simulink model "control_filtro_pq_lspyc"  (R2017b)
settings: Solver=ode1  StartTime=0.0  StopTime=0.5  FixedStep=Ts  MaxStep=1e-4  RelTol=1e-3
InitFcn:
  | GlobalParam
values from neighbouring files (symbols this model uses):
  APFon = 0.025    [GlobalParam.m]
  Cdc = 2480e-6    (= 0.00248)    [GlobalParam.m]
  fc = 18000    [GlobalParam.m]
  fe = 50    [GlobalParam.m]
  Ideal = 0    [GlobalParam.m]
  Lf = 0.01    [GlobalParam.m]
  LL = 0.055462    [GlobalParam.m]
  nc = 3    [GlobalParam.m]
  NLLon = 6    [GlobalParam.m]
  Rf = 0.35    [GlobalParam.m]
  RL = 23.232    [GlobalParam.m]
  RLon = 0.0    (= 0)    [GlobalParam.m]
  teta_a = 0    [GlobalParam.m]
  teta_b = -120    [GlobalParam.m]
  teta_c = 120    [GlobalParam.m]
  Tm = 1/fm    (= 5.55555555556e-05)    [GlobalParam.m]
  Ts = 5e-6    (= 5e-06)    [GlobalParam.m]
  Vdc = 63    [GlobalParam.m]
  Vs = 120*sqrt(2)    [GlobalParam.m]
undefined symbols (not defined in the file or in its folder): magnitude
libraries: powerlib x113, simulink x9, powerlib_meascontrol x6, powerlib_extras x5
(part 1 of 2)
settings Model: Creator=user  LastModifiedBy=user
settings OptimizationCC: LifeSpan=inf
settings DebuggingCC: SFExecutionAtInitializationDiag=none
settings CodeAppCC: StateflowObjectComments=on
settings SimscapeCC: SimscapeNormalizeSystem=off

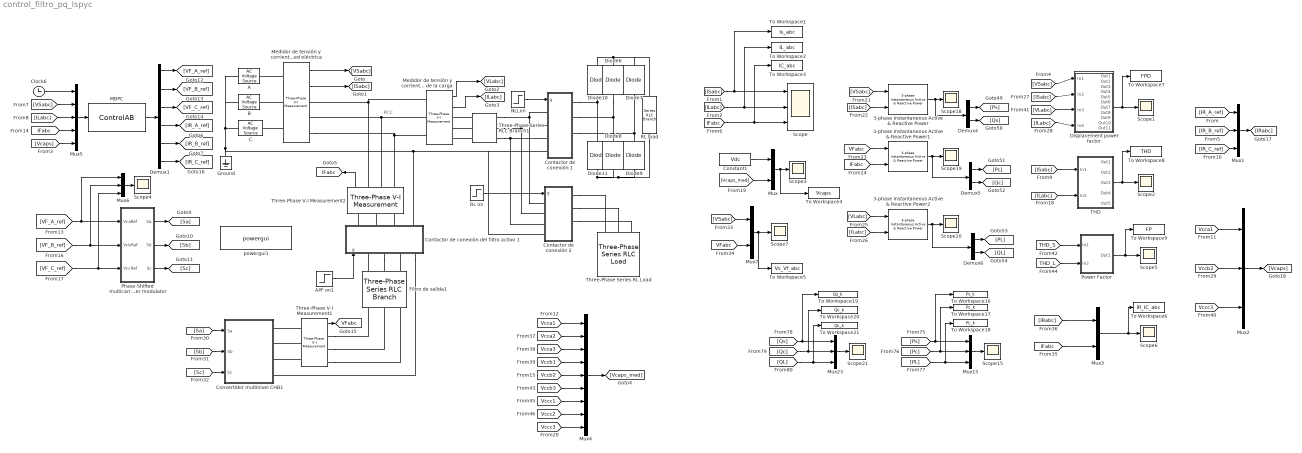
== system control_filtro_pq_lspyc ==
  note: PCC
  " RL load" : powerlib/Elements/Series RLC Branch  LConnTagsString=__new0  RConnTagsString=__new0  BranchType=RL  Resistance=RL*6  Inductance=LL/6  SetiL0=off  InitialCurrent=0  Capacitance=1e-6  Setx0=off  InitialVoltage=0  Measurements=None
  3-phase Instantaneous Active & Reactive Power : powerlib_extras/Measurements/3-phase  Instantaneous  Active & Reactive Power
  3-phase Instantaneous Active & Reactive Power1 : powerlib_extras/Measurements/3-phase  Instantaneous  Active & Reactive Power
  3-phase Instantaneous Active & Reactive Power2 : powerlib_extras/Measurements/3-phase  Instantaneous  Active & Reactive Power
  "A " : powerlib/Electrical Sources/AC Voltage Source  Amplitude=Vs  Phase=teta_a  Frequency=fe  SampleTime=0  Measurements=None  BusType=swing  Pref=10e3  Qref=0  Qmin=-inf  Qmax=+inf
  APF on1 : Step  Time=APFon  SampleTime=0
  "B " : powerlib/Electrical Sources/AC Voltage Source  Amplitude=Vs  Phase=teta_b  Frequency=fe  SampleTime=0  Measurements=None  BusType=swing  Pref=10e3  Qref=0  Qmin=-inf  Qmax=+inf
  "C " : powerlib/Electrical Sources/AC Voltage Source  Amplitude=Vs  Phase=teta_c  Frequency=fe  SampleTime=0  Measurements=None  BusType=swing  Pref=10e3  Qref=0  Qmin=-inf  Qmax=+inf
  Clock6 : Clock
  Constant1 : Constant  Value=Vdc
  Contactor de conexión del filtro activo 1 : Subsystem
  Contactor de conexión 1 : Subsystem
  "Contactor de conexión 2 " : Subsystem
  Convertidor multinivel CHB1 : Subsystem
  Demux1 : Demux  Outputs=6
  Demux4 : Demux  Outputs=2
  Demux5 : Demux  Outputs=2
  Demux6 : Demux  Outputs=2
  Diode{6..11} (6 alike) : powerlib/Power Electronics/Diode  Ron=0.001  Lon=0  Vf=0  IC=0  UseSnubber=off  Rs=500  Cs=250e-9  Measurements=off
  Displacement power factor : Subsystem
  Filtro de salida1 : powerlib/Elements/Three-Phase Series RLC Branch  LConnTagsString=A|B|C  RConnTagsString=A|B|C  BranchType=RL  Resistance=Rf  Inductance=Lf  Capacitance=1e-6  Measurements=None
  Ground : powerlib/Elements/Ground  LConnTagsString=a
  MBPC : MATLABFcn  MATLABFcn=ControlAB  OutputDimensions=6
  Medidor de tensión y corriente de la red eléctrica : powerlib/Measurements/Three-Phase V-I Measurement  VoltageMeasurement=phase-to-ground  SetLabelV=off  LabelV=Vabc  Vpu=off  VpuLL=off  CurrentMeasurement=yes  SetLabelI=off  LabelI=Iabc  Ipu=off  Pbase=100e6  Vbase=500e3  OutputType=Complex  PhasorSimulation=off  PSBequivalent=0
  "Medidor de tensión y corriente de la carga " : powerlib/Measurements/Three-Phase V-I Measurement  VoltageMeasurement=phase-to-ground  SetLabelV=off  LabelV=Vabc  Vpu=off  VpuLL=off  CurrentMeasurement=yes  SetLabelI=off  LabelI=Iabc  Ipu=off  Pbase=100e6  Vbase=500e3  OutputType=Complex  PhasorSimulation=off  PSBequivalent=0
  Mux : Mux  Inputs=2
  Mux{1..2,6,15,23} (5 alike) : Mux  Inputs=3
  Mux3 : Mux  Inputs=2
  Mux4 : Mux  Inputs=9
  Mux5 : Mux  Inputs=5
  Mux7 : Mux  Inputs=2
  "NLLon " : Step  Time=NLLon  SampleTime=0
  Phase-Shifted multicarrier modulator : Subsystem
  "Power Factor " : Subsystem
  "RL on " : Step  Time=RLon  SampleTime=0
  Scope : Scope  NumInputPorts=3
  Scope{1..7,15,18..21} (12 alike) : Scope
  "THD " : Subsystem
  Three-Phase Series RL Load : powerlib/Elements/Three-Phase Series RLC Load  LConnTagsString=A|B|C  Configuration=Y (grounded)  NominalVoltage=120  Vabc=[120 120 120]  Vabcp=[1e3 1e3 1e3]  NominalFrequency=50  UnbalancedPower=on  ActivePower=350/3  InductivePower=833/3  CapacitivePower=0  Pabc=[280 280 280]  QLabc=[200 200 200]  QCabc=[0 0 0]  Pabcp=[10e3 9e3 11e3]  QLabcp=[100 90 110]  QCabcp=[100 90 110]  Measurements=None  LoadType=constant Z
  Three-Phase Series RLC Branch1 : powerlib/Elements/Three-Phase Series RLC Branch  LConnTagsString=A|B|C  RConnTagsString=A|B|C  BranchType=RL  Resistance=0.1  Inductance=0.001  Capacitance=1e-6  Measurements=None
  Three-Phase V-I Measurement1 : powerlib/Measurements/Three-Phase V-I Measurement  VoltageMeasurement=phase-to-ground  SetLabelV=off  LabelV=Vabc  Vpu=off  VpuLL=off  CurrentMeasurement=no  SetLabelI=off  LabelI=Iabc  Ipu=off  Pbase=100e6  Vbase=500e3  OutputType=Complex  PhasorSimulation=off  PSBequivalent=0
  Three-Phase V-I Measurement2 : powerlib/Measurements/Three-Phase V-I Measurement  VoltageMeasurement=no  SetLabelV=off  LabelV=Vabc  Vpu=off  VpuLL=off  CurrentMeasurement=yes  SetLabelI=off  LabelI=Iabc  Ipu=off  Pbase=100e6  Vbase=500e3  OutputType=Complex  PhasorSimulation=off  PSBequivalent=0
  To Workspace1 : ToWorkspace  VariableName=Is_abc  SaveFormat=Timeseries  SampleTime=-1
  To Workspace16 : ToWorkspace  VariableName=Ps_k  SaveFormat=Timeseries  SampleTime=-1
  To Workspace17 : ToWorkspace  VariableName=Pc_k  SaveFormat=Timeseries  SampleTime=-1
  To Workspace18 : ToWorkspace  VariableName=PL_k  SaveFormat=Timeseries  SampleTime=-1
  To Workspace19 : ToWorkspace  VariableName=Qs_k  SaveFormat=Timeseries  SampleTime=-1
  To Workspace2 : ToWorkspace  VariableName=IL_abc  SaveFormat=Timeseries  SampleTime=-1
  To Workspace20 : ToWorkspace  VariableName=Qc_k  SaveFormat=Timeseries  SampleTime=-1
  To Workspace21 : ToWorkspace  VariableName=QL_k  SaveFormat=Timeseries  SampleTime=-1
  To Workspace3 : ToWorkspace  VariableName=IC_abc  SaveFormat=Timeseries  SampleTime=-1
  To Workspace4 : ToWorkspace  VariableName=Vcaps  SaveFormat=Timeseries  SampleTime=-1
  To Workspace5 : ToWorkspace  VariableName=Vs_Vf_abc  SaveFormat=Timeseries  SampleTime=-1
  To Workspace6 : ToWorkspace  VariableName=IR_IC_abc  SaveFormat=Timeseries  SampleTime=-1
  To Workspace7 : ToWorkspace  VariableName=FPD  SaveFormat=Timeseries  SampleTime=-1
  To Workspace8 : ToWorkspace  VariableName=THD  SaveFormat=Timeseries  SampleTime=-1
  To Workspace9 : ToWorkspace  VariableName=FP  SaveFormat=Timeseries  SampleTime=-1
  powergui1 : powerlib/powergui  Priority=1  SimulationMode=Discrete  SampleTime=Ts  frequency=60  Iterations=50  frequencyindice=50  Pbase=100e6  ErrMax=1e-4  UnitsV=kV  UnitsW=MW  buscounter=0  FunctionMessages=off  echomessages=off  EnableUseOfTLC=off  CurrentSourceSwitches=off  DisableSnubberDevices=off  DisableRonSwitches=off  DisableVfSwitches=off  DisplayEquations=off  SolverType=Tustin/Backward Euler (TBE)  Interpol=off  ExternalGateDelay=off  methode=off  Ts=100  x0status=blocks  SPID=on  SwTol=0  HookPort=off  RestoreLinks=warning  ResistiveCurrentMeasurement=off  Frange=[0:2:500]  Ylog=off  Xlog=on  ShowGrid=off  save=off  variable=ZData  structure=ScopeData  ZoomFFT=off  StartTime=0.3  cycles=15  DisplayStyle=1  fundamental=50  FreqAxis=on  MaxFrequency=1500  frequencyindicesteady=1  RmsSteady=1  display=off
  tag scope: IFabc=global, VFabc=global
  wires:
  Medidor de tensión y corriente de la red eléctrica/1 -> [VSabc]
  Medidor de tensión y corriente de la red eléctrica/2 -> [ISabc]
  "Medidor de tensión y corriente de la carga "/2 -> [ILabc]
  [ILabc] -> To Workspace2/1, Scope/2
  Three-Phase V-I Measurement2/1 -> [IFabc]
  Mux5/1 -> MBPC/1
  Clock6/1 -> Mux5/1
  [IFabc] -> To Workspace3/1, Scope/3
  [ISabc] -> To Workspace1/1, Scope/1
  Constant1/1 -> Mux/1
  Mux/1 -> To Workspace4/1, Scope3/1
  Mux6/1 -> Scope4/1
  Phase-Shifted multicarrier modulator/3(Sc) -> [Sc]
  Phase-Shifted multicarrier modulator/1(Sa) -> [Sa]
  [VF_B_ref] -> Mux6/2, Phase-Shifted multicarrier modulator/2(VcbRef)
  [VF_C_ref] -> Mux6/3, Phase-Shifted multicarrier modulator/3(VccRef)
  [VF_A_ref] -> Mux6/1, Phase-Shifted multicarrier modulator/1(VcaRef)
  Phase-Shifted multicarrier modulator/2(Sb) -> [Sb]
  Demux1/1 -> [VF_A_ref]
  Demux1/2 -> [VF_B_ref]
  Demux1/3 -> [VF_C_ref]
  Three-Phase V-I Measurement1/1 -> [VFabc]
  [IFabc] -> Mux3/2
  [IRabc] -> Mux3/1
  [VFabc] -> Mux7/2
  [VSabc] -> Mux7/1
  [Sc] -> Convertidor multinivel CHB1/3(Sc)
  [Sb] -> Convertidor multinivel CHB1/2(Sb)
  Mux3/1 -> To Workspace6/1, Scope6/1
  APF on1/1 -> Contactor de conexión del filtro activo 1/1(g)
  [Sa] -> Convertidor multinivel CHB1/1(Sa)
  Mux7/1 -> To Workspace5/1, Scope7/1
  [Vcaps] -> Mux5/5
  [IFabc] -> Mux5/4
  [ILabc] -> Mux5/3
  [VSabc] -> Mux5/2
  Demux1/4 -> [IR_A_ref]
  Demux1/5 -> [IR_B_ref]
  Demux1/6 -> [IR_C_ref]
  Mux1/1 -> [IRabc]
  [IR_A_ref] -> Mux1/1
  [IR_B_ref] -> Mux1/2
  [IR_C_ref] -> Mux1/3
  Mux2/1 -> [Vcaps]
  [Vcaps_med] -> Mux/2
  MBPC/1 -> Demux1/1
  "RL on "/1 -> "Contactor de conexión 2 "/1(g)
  3-phase Instantaneous Active & Reactive Power/1 -> Scope18/1, Demux4/1
  [VSabc] -> 3-phase Instantaneous Active & Reactive Power/1
  Demux4/2 -> [Qs]
  [ISabc] -> 3-phase Instantaneous Active & Reactive Power/2
  Demux4/1 -> [Ps]
  [IFabc] -> 3-phase Instantaneous Active & Reactive Power1/2
  3-phase Instantaneous Active & Reactive Power1/1 -> Scope19/1, Demux5/1
  [VFabc] -> 3-phase Instantaneous Active & Reactive Power1/1
  Demux5/1 -> [Pc]
  Demux5/2 -> [Qc]
  [VLabc] -> 3-phase Instantaneous Active & Reactive Power2/1
  [ILabc] -> 3-phase Instantaneous Active & Reactive Power2/2
  3-phase Instantaneous Active & Reactive Power2/1 -> Scope20/1, Demux6/1
  Demux6/1 -> [PL]
  Demux6/2 -> [QL]
  Mux15/1 -> Scope15/1
  [Qc] -> Mux23/2, To Workspace20/1
  [PL] -> Mux15/3, To Workspace18/1
  [Ps] -> Mux15/1, To Workspace16/1
  [Pc] -> Mux15/2, To Workspace17/1
  [QL] -> Mux23/3, To Workspace21/1
  Mux23/1 -> Scope21/1
  [Qs] -> Mux23/1, To Workspace19/1
  "Medidor de tensión y corriente de la carga "/1 -> [VLabc]
  "NLLon "/1 -> Contactor de conexión 1/1(g)
  "Power Factor "/1(Out1) -> Scope5/1, To Workspace9/1
  [THD_S] -> "Power Factor "/1(In1)
  [THD_L] -> "Power Factor "/2(In2)
  "THD "/3(Out3) -> Scope2/1, To Workspace8/1
  [ISabc] -> "THD "/1(In1)
  [ILabc] -> "THD "/2(In2)
  Displacement power factor/7(Out7) -> To Workspace7/1, Scope1/1
  [VSabc] -> Displacement power factor/1(In1)
  [ISabc] -> Displacement power factor/2(In2)
  [VLabc] -> Displacement power factor/3(In3)
  [ILabc] -> Displacement power factor/4(In4)
  [Vccc3] -> Mux2/3
  [Vccb2] -> Mux2/2
  [Vcca1] -> Mux2/1
  Mux4/1 -> [Vcaps_med]
  [Vcca1] -> Mux4/1
  [Vcca2] -> Mux4/2
  [Vcca3] -> Mux4/3
  [Vccb1] -> Mux4/4
  [Vccb2] -> Mux4/5
  [Vccb3] -> Mux4/6
  [Vccc1] -> Mux4/7
  [Vccc3] -> Mux4/9
  [Vccc2] -> Mux4/8
  connections:
  Contactor de conexión del filtro activo 1/RConn4 -- Contactor de conexión 1/LConn4 -- "Contactor de conexión 2 "/LConn4 -- "C "/LConn1 -- "A "/LConn1 -- "B "/LConn1 -- Ground/LConn1
  "Medidor de tensión y corriente de la carga "/LConn1 -- Three-Phase V-I Measurement2/RConn1 -- Medidor de tensión y corriente de la red eléctrica/RConn1
  "Medidor de tensión y corriente de la carga "/LConn2 -- Three-Phase V-I Measurement2/RConn2 -- Medidor de tensión y corriente de la red eléctrica/RConn2
  Medidor de tensión y corriente de la red eléctrica/RConn3 -- Three-Phase V-I Measurement2/RConn3 -- "Medidor de tensión y corriente de la carga "/LConn3
  Filtro de salida1/RConn1 -- Contactor de conexión del filtro activo 1/LConn1
  Three-Phase V-I Measurement1/LConn3 -- Convertidor multinivel CHB1/RConn3
  Three-Phase V-I Measurement1/LConn1 -- Convertidor multinivel CHB1/RConn1
  Three-Phase V-I Measurement1/RConn1 -- Filtro de salida1/LConn1
  Contactor de conexión del filtro activo 1/LConn2 -- Filtro de salida1/RConn2
  Three-Phase V-I Measurement1/LConn2 -- Convertidor multinivel CHB1/RConn2
  Filtro de salida1/RConn3 -- Contactor de conexión del filtro activo 1/LConn3
  Contactor de conexión del filtro activo 1/LConn4 -- Convertidor multinivel CHB1/RConn4
  Three-Phase V-I Measurement1/RConn3 -- Filtro de salida1/LConn3
  Three-Phase V-I Measurement1/RConn2 -- Filtro de salida1/LConn2
  Contactor de conexión del filtro activo 1/RConn1 -- Three-Phase V-I Measurement2/LConn1
  Contactor de conexión del filtro activo 1/RConn2 -- Three-Phase V-I Measurement2/LConn2
  Contactor de conexión del filtro activo 1/RConn3 -- Three-Phase V-I Measurement2/LConn3
  Medidor de tensión y corriente de la red eléctrica/LConn3 -- "C "/RConn1
  Medidor de tensión y corriente de la red eléctrica/LConn2 -- "B "/RConn1
  Medidor de tensión y corriente de la red eléctrica/LConn1 -- "A "/RConn1
  "Contactor de conexión 2 "/RConn1 -- Three-Phase Series RL Load/LConn1
  "Contactor de conexión 2 "/RConn2 -- Three-Phase Series RL Load/LConn2
  "Contactor de conexión 2 "/RConn3 -- Three-Phase Series RL Load/LConn3
  Contactor de conexión 1/LConn1 -- Three-Phase Series RLC Branch1/RConn1 -- "Contactor de conexión 2 "/LConn1
  Contactor de conexión 1/LConn2 -- Three-Phase Series RLC Branch1/RConn2 -- "Contactor de conexión 2 "/LConn2
  Contactor de conexión 1/LConn3 -- Three-Phase Series RLC Branch1/RConn3 -- "Contactor de conexión 2 "/LConn3
  Three-Phase Series RLC Branch1/LConn3 -- "Medidor de tensión y corriente de la carga "/RConn3
  Three-Phase Series RLC Branch1/LConn2 -- "Medidor de tensión y corriente de la carga "/RConn2
  Three-Phase Series RLC Branch1/LConn1 -- "Medidor de tensión y corriente de la carga "/RConn1
  Diode10/LConn1 -- Contactor de conexión 1/RConn1 -- Diode11/RConn1
  Diode6/RConn1 -- " RL load"/LConn1 -- Diode7/RConn1 -- Diode10/RConn1
  Diode9/RConn1 -- Contactor de conexión 1/RConn3 -- Diode7/LConn1
  Diode6/LConn1 -- Contactor de conexión 1/RConn2 -- Diode8/RConn1
  Diode11/LConn1 -- " RL load"/RConn1 -- Diode9/LConn1 -- Diode8/LConn1

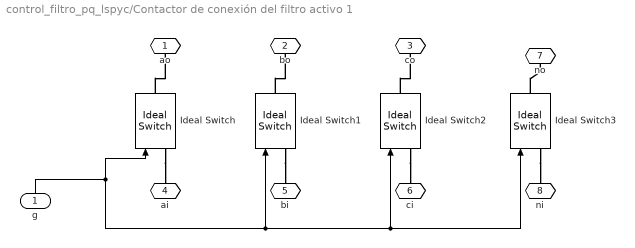
== system control_filtro_pq_lspyc/Contactor de conexión del filtro activo 1 ==
  g : Inport
  Ideal Switch{,1..3} (4 alike) : powerlib/Power Electronics/Ideal Switch  Ron=0.001  Lon=0  IC=0  Rs=1e5  Cs=inf  Measurements=off
  ao : PMIOPort  Port=1  Side=Right
  bo : PMIOPort  Port=2  Side=Right
  co : PMIOPort  Port=3  Side=Right
  ai : PMIOPort  Port=4  Side=Left
  bi : PMIOPort  Port=5  Side=Left
  ci : PMIOPort  Port=6  Side=Left
  no : PMIOPort  Port=7  Side=Left
  ni : PMIOPort  Port=8  Side=Right
  wires:
  g/1 -> Ideal Switch3/1, Ideal Switch2/1, Ideal Switch1/1, Ideal Switch/1
  connections:
  Ideal Switch1/RConn1 -- bo/RConn1
  Ideal Switch1/LConn1 -- bi/RConn1
  Ideal Switch/RConn1 -- ao/RConn1
  Ideal Switch2/RConn1 -- co/RConn1
  Ideal Switch2/LConn1 -- ci/RConn1
  Ideal Switch/LConn1 -- ai/RConn1
  Ideal Switch3/LConn1 -- ni/RConn1
  Ideal Switch3/RConn1 -- no/RConn1

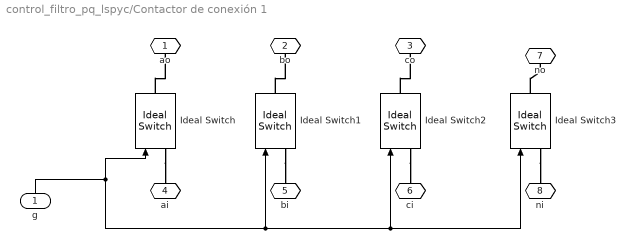
== system control_filtro_pq_lspyc/Contactor de conexión 1 ==
  g : Inport
  Ideal Switch{,1..3} (4 alike) : powerlib/Power Electronics/Ideal Switch  Ron=0.001  Lon=0  IC=0  Rs=1e5  Cs=inf  Measurements=off
  ao : PMIOPort  Port=1  Side=Right
  bo : PMIOPort  Port=2  Side=Right
  co : PMIOPort  Port=3  Side=Right
  ai : PMIOPort  Port=4  Side=Left
  bi : PMIOPort  Port=5  Side=Left
  ci : PMIOPort  Port=6  Side=Left
  no : PMIOPort  Port=7  Side=Left
  ni : PMIOPort  Port=8  Side=Right
  wires:
  g/1 -> Ideal Switch3/1, Ideal Switch2/1, Ideal Switch1/1, Ideal Switch/1
  connections:
  Ideal Switch1/RConn1 -- bo/RConn1
  Ideal Switch1/LConn1 -- bi/RConn1
  Ideal Switch/RConn1 -- ao/RConn1
  Ideal Switch2/RConn1 -- co/RConn1
  Ideal Switch2/LConn1 -- ci/RConn1
  Ideal Switch/LConn1 -- ai/RConn1
  Ideal Switch3/LConn1 -- ni/RConn1
  Ideal Switch3/RConn1 -- no/RConn1

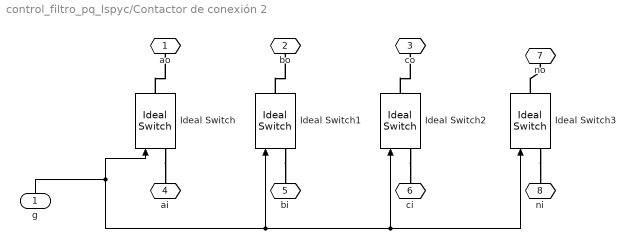
== system control_filtro_pq_lspyc/Contactor de conexión 2  ==
  g : Inport
  Ideal Switch{,1..3} (4 alike) : powerlib/Power Electronics/Ideal Switch  Ron=0.001  Lon=0  IC=0  Rs=1e5  Cs=inf  Measurements=off
  ao : PMIOPort  Port=1  Side=Right
  bo : PMIOPort  Port=2  Side=Right
  co : PMIOPort  Port=3  Side=Right
  ai : PMIOPort  Port=4  Side=Left
  bi : PMIOPort  Port=5  Side=Left
  ci : PMIOPort  Port=6  Side=Left
  no : PMIOPort  Port=7  Side=Left
  ni : PMIOPort  Port=8  Side=Right
  wires:
  g/1 -> Ideal Switch3/1, Ideal Switch2/1, Ideal Switch1/1, Ideal Switch/1
  connections:
  Ideal Switch1/RConn1 -- bo/RConn1
  Ideal Switch1/LConn1 -- bi/RConn1
  Ideal Switch/RConn1 -- ao/RConn1
  Ideal Switch2/RConn1 -- co/RConn1
  Ideal Switch2/LConn1 -- ci/RConn1
  Ideal Switch/LConn1 -- ai/RConn1
  Ideal Switch3/LConn1 -- ni/RConn1
  Ideal Switch3/RConn1 -- no/RConn1

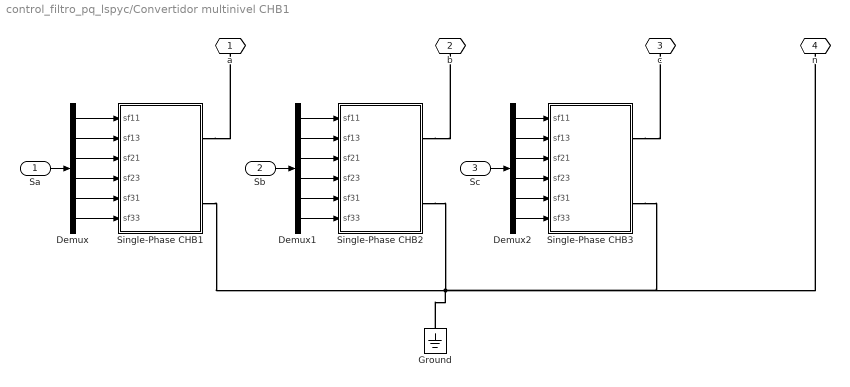
== system control_filtro_pq_lspyc/Convertidor multinivel CHB1 ==
  Sa : Inport
  Sb : Inport  Port=2
  Sc : Inport  Port=3
  Demux : Demux  Outputs=6
  Demux1 : Demux  Outputs=6
  Demux2 : Demux  Outputs=6
  Ground : powerlib/Elements/Ground  LConnTagsString=a
  Single-Phase CHB1 : Subsystem
  Single-Phase CHB2 : Subsystem
  Single-Phase CHB3 : Subsystem
  a : PMIOPort  Port=1  Side=Right
  b : PMIOPort  Port=2  Side=Right
  c : PMIOPort  Port=3  Side=Right
  n : PMIOPort  Port=4  Side=Right
  wires:
  Demux/4 -> Single-Phase CHB1/4(sf23)
  Demux/6 -> Single-Phase CHB1/6(sf33)
  Demux/3 -> Single-Phase CHB1/3(sf21)
  Demux/2 -> Single-Phase CHB1/2(sf13)
  Demux/1 -> Single-Phase CHB1/1(sf11)
  Demux1/3 -> Single-Phase CHB2/3(sf21)
  Sa/1 -> Demux/1
  Sb/1 -> Demux1/1
  Sc/1 -> Demux2/1
  Demux2/1 -> Single-Phase CHB3/1(sf11)
  Demux1/1 -> Single-Phase CHB2/1(sf11)
  Demux1/6 -> Single-Phase CHB2/6(sf33)
  Demux2/6 -> Single-Phase CHB3/6(sf33)
  Demux/5 -> Single-Phase CHB1/5(sf31)
  Demux1/2 -> Single-Phase CHB2/2(sf13)
  Demux2/5 -> Single-Phase CHB3/5(sf31)
  Demux1/4 -> Single-Phase CHB2/4(sf23)
  Demux2/4 -> Single-Phase CHB3/4(sf23)
  Demux1/5 -> Single-Phase CHB2/5(sf31)
  Demux2/3 -> Single-Phase CHB3/3(sf21)
  Demux2/2 -> Single-Phase CHB3/2(sf13)
  connections:
  Single-Phase CHB2/RConn1 -- b/RConn1
  Single-Phase CHB1/RConn2 -- Ground/LConn1 -- Single-Phase CHB2/RConn2 -- Single-Phase CHB3/RConn2 -- n/RConn1
  Single-Phase CHB1/RConn1 -- a/RConn1
  Single-Phase CHB3/RConn1 -- c/RConn1

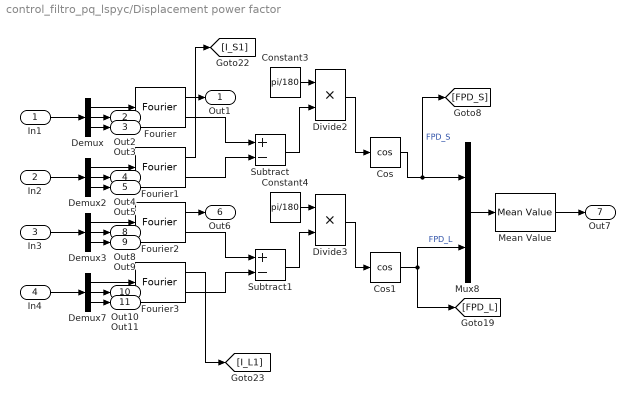
== system control_filtro_pq_lspyc/Displacement power factor ==
  In1 : Inport
  In2 : Inport  Port=2
  In3 : Inport  Port=3
  In4 : Inport  Port=4
  Constant3 : Constant  Value=pi/180
  Constant4 : Constant  Value=pi/180
  Cos : Trigonometry  Operator=cos
  Cos1 : Trigonometry  Operator=cos
  Demux{,2..3,7} (4 alike) : Demux  Outputs=3
  Divide2 : Product  Inputs=**
  Divide3 : Product  Inputs=**
  Fourier{,1..3} (4 alike) : powerlib_meascontrol/Measurements/Fourier  Freq=60  n=1  InInit=[0, 0]  Ts=0
      settings: SourceProductName=Simscape Power Systems
  Mean Value : powerlib_extras/Measurements/Mean Value  Period=1/100
  Mux8 : Mux  Inputs=2
  Subtract : Sum  Inputs=+-
  Subtract1 : Sum  Inputs=+-
  Out1 : Outport
  Out2 : Outport  Port=2
  Out3 : Outport  Port=3
  Out4 : Outport  Port=4
  Out5 : Outport  Port=5
  Out6 : Outport  Port=6
  Out7 : Outport  Port=7
  Out8 : Outport  Port=8
  Out9 : Outport  Port=9
  Out10 : Outport  Port=10
  Out11 : Outport  Port=11
  wires:
  Demux/3 -> Out3/1
  Fourier2/1 -> Out6/1
  Demux/2 -> Out2/1
  Demux7/2 -> Out10/1
  Demux3/2 -> Out8/1
  Fourier/1 -> Out1/1
  Demux7/3 -> Out11/1
  Demux3/3 -> Out9/1
  Fourier3/2 -> Subtract1/2
  Mux8/1 -> Mean Value/1
  Demux2/1 -> Fourier1/1
  In1/1 -> Demux/1
  Constant3/1 -> Divide2/1
  Fourier1/1 -> [I_S1]
  Subtract/1 -> Divide2/2
  Fourier2/2 -> Subtract1/1
  Cos/1 -> Mux8/1, [FPD_S]  "FPD_S"
  Demux/1 -> Fourier/1
  Mean Value/1 -> Out7/1
  Demux3/1 -> Fourier2/1
  Divide3/1 -> Cos1/1
  Fourier1/2 -> Subtract/2
  Constant4/1 -> Divide3/1
  In2/1 -> Demux2/1
  Fourier/2 -> Subtract/1
  Demux7/1 -> Fourier3/1
  Cos1/1 -> Mux8/2, [FPD_L]  "FPD_L"
  In3/1 -> Demux3/1
  In4/1 -> Demux7/1
  Subtract1/1 -> Divide3/2
  Fourier3/1 -> [I_L1]
  Divide2/1 -> Cos/1
  Demux2/2 -> Out4/1
  Demux2/3 -> Out5/1

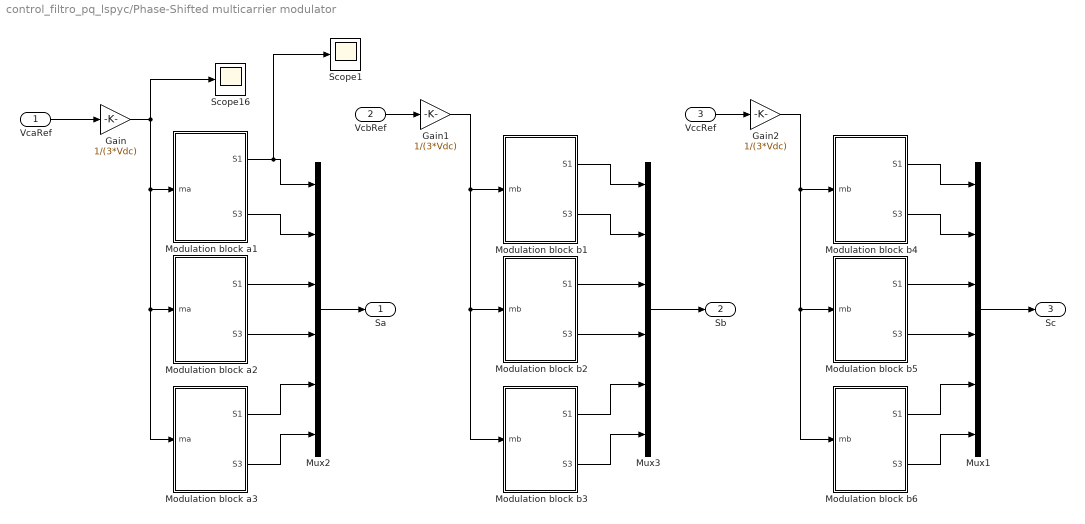
== system control_filtro_pq_lspyc/Phase-Shifted multicarrier modulator ==
  VcaRef : Inport
  VcbRef : Inport  Port=2
  VccRef : Inport  Port=3
  Gain : Gain  Gain=1/(3*Vdc)
  Gain1 : Gain  Gain=1/(3*Vdc)
  Gain2 : Gain  Gain=1/(3*Vdc)
  Modulation block a1 : Subsystem
  Modulation block a2 : Subsystem
  Modulation block a3 : Subsystem
  Modulation block b1 : Subsystem
  Modulation block b2 : Subsystem
  Modulation block b3 : Subsystem
  Modulation block b4 : Subsystem
  Modulation block b5 : Subsystem
  Modulation block b6 : Subsystem
  Mux1 : Mux  Inputs=6
  Mux2 : Mux  Inputs=6
  Mux3 : Mux  Inputs=6
  Scope1 : Scope
  Scope16 : Scope
  Sa : Outport
  Sb : Outport  Port=2
  Sc : Outport  Port=3
  wires:
  Gain1/1 -> Modulation block b1/1(mb), Modulation block b2/1(mb), Modulation block b3/1(mb)
  Gain/1 -> Modulation block a1/1(ma), Modulation block a3/1(ma), Modulation block a2/1(ma), Scope16/1
  Modulation block a2/2(S3) -> Mux2/4
  Modulation block a2/1(S1) -> Mux2/3
  Modulation block a3/1(S1) -> Mux2/5
  Modulation block a3/2(S3) -> Mux2/6
  Modulation block a1/2(S3) -> Mux2/2
  Mux2/1 -> Sa/1
  Modulation block b2/2(S3) -> Mux3/4
  Modulation block b3/1(S1) -> Mux3/5
  Modulation block b3/2(S3) -> Mux3/6
  Modulation block b2/1(S1) -> Mux3/3
  Modulation block b1/2(S3) -> Mux3/2
  Modulation block b1/1(S1) -> Mux3/1
  Mux3/1 -> Sb/1
  VcbRef/1 -> Gain1/1
  VccRef/1 -> Gain2/1
  VcaRef/1 -> Gain/1
  Modulation block a1/1(S1) -> Scope1/1, Mux2/1
  Gain2/1 -> Modulation block b4/1(mb), Modulation block b5/1(mb), Modulation block b6/1(mb)
  Modulation block b4/2(S3) -> Mux1/2
  Modulation block b4/1(S1) -> Mux1/1
  Mux1/1 -> Sc/1
  Modulation block b5/1(S1) -> Mux1/3
  Modulation block b6/2(S3) -> Mux1/6
  Modulation block b6/1(S1) -> Mux1/5
  Modulation block b5/2(S3) -> Mux1/4

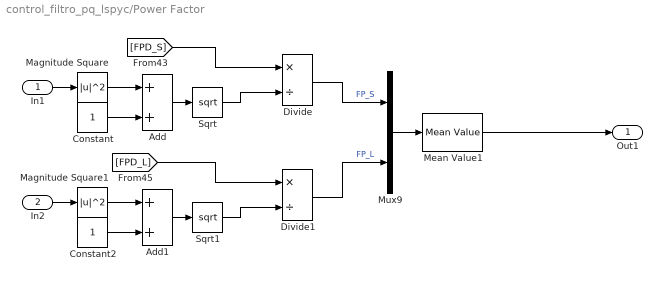
== system control_filtro_pq_lspyc/Power Factor  ==
  In1 : Inport
  In2 : Inport  Port=2
  Add : Sum
  Add1 : Sum
  Constant : Constant
  Constant2 : Constant
  Divide : Product  Inputs=*/
  Divide1 : Product  Inputs=*/
  Magnitude Square : Math  Operator=magnitude^2  RndMeth=Zero  SaturateOnIntegerOverflow=on
  Magnitude Square1 : Math  Operator=magnitude^2  RndMeth=Zero  SaturateOnIntegerOverflow=on
  Mean Value1 : powerlib_extras/Measurements/Mean Value  Period=1/100
  Mux9 : Mux  Inputs=2
  Sqrt : Sqrt  SaturateOnIntegerOverflow=on
  Sqrt1 : Sqrt  SaturateOnIntegerOverflow=on
  Out1 : Outport
  wires:
  In1/1 -> Magnitude Square/1
  Magnitude Square/1 -> Add/1
  Divide1/1 -> Mux9/2  "FP_L"
  Constant/1 -> Add/2
  Mux9/1 -> Mean Value1/1
  Sqrt/1 -> Divide/2
  [FPD_L] -> Divide1/1
  [FPD_S] -> Divide/1
  Add1/1 -> Sqrt1/1
  Add/1 -> Sqrt/1
  In2/1 -> Magnitude Square1/1
  Constant2/1 -> Add1/2
  Sqrt1/1 -> Divide1/2
  Magnitude Square1/1 -> Add1/1
  Divide/1 -> Mux9/1  "FP_S"
  Mean Value1/1 -> Out1/1

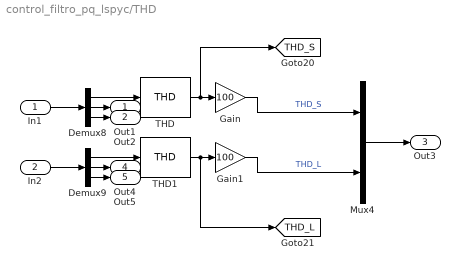
== system control_filtro_pq_lspyc/THD  ==
  In1 : Inport
  In2 : Inport  Port=2
  Demux8 : Demux  Outputs=3
  Demux9 : Demux  Outputs=3
  Gain : Gain  Gain=100
  Gain1 : Gain  Gain=100
  Mux4 : Mux  Inputs=2
  THD : powerlib_meascontrol/Measurements/THD  Freq=50  Ts=Ts
  THD1 : powerlib_meascontrol/Measurements/THD  Freq=50  Ts=Ts
  Out1 : Outport
  Out2 : Outport  Port=2
  Out3 : Outport  Port=3
  Out4 : Outport  Port=4
  Out5 : Outport  Port=5
  tag scope: THD_L=global, THD_S=global
  wires:
  Demux8/1 -> THD/1
  Gain1/1 -> Mux4/2  "THD_L"
  Mux4/1 -> Out3/1
  Gain/1 -> Mux4/1  "THD_S"
  In2/1 -> Demux9/1
  THD1/1 -> [THD_L], Gain1/1
  Demux9/1 -> THD1/1
  In1/1 -> Demux8/1
  THD/1 -> [THD_S], Gain/1
  Demux8/3 -> Out2/1
  Demux8/2 -> Out1/1
  Demux9/2 -> Out4/1
  Demux9/3 -> Out5/1

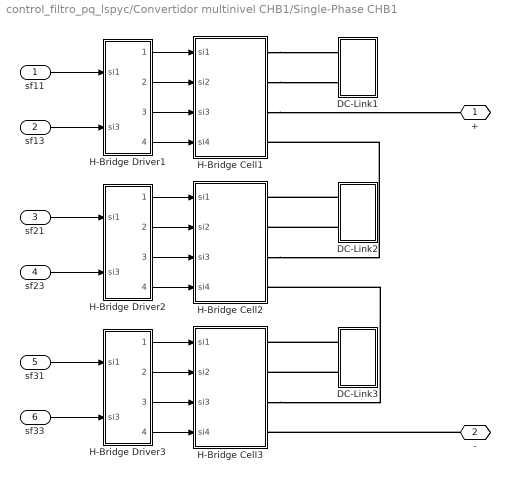
== system control_filtro_pq_lspyc/Convertidor multinivel CHB1/Single-Phase CHB1 ==
  sf11 : Inport
  sf13 : Inport  Port=2
  sf21 : Inport  Port=3
  sf23 : Inport  Port=4
  sf31 : Inport  Port=5
  sf33 : Inport  Port=6
  DC-Link1 : Subsystem
  DC-Link2 : Subsystem
  DC-Link3 : Subsystem
  H-Bridge Cell1 : Subsystem
  H-Bridge Cell2 : Subsystem
  H-Bridge Cell3 : Subsystem
  H-Bridge Driver1 : Subsystem
  H-Bridge Driver2 : Subsystem
  H-Bridge Driver3 : Subsystem
  + : PMIOPort  Port=1  Side=Right
  - : PMIOPort  Port=2  Side=Right
  wires:
  H-Bridge Driver2/1(1) -> H-Bridge Cell2/1(si1)
  H-Bridge Driver2/3(3) -> H-Bridge Cell2/3(si3)
  H-Bridge Driver2/2(2) -> H-Bridge Cell2/2(si2)
  H-Bridge Driver2/4(4) -> H-Bridge Cell2/4(si4)
  H-Bridge Driver1/1(1) -> H-Bridge Cell1/1(si1)
  H-Bridge Driver1/2(2) -> H-Bridge Cell1/2(si2)
  H-Bridge Driver1/3(3) -> H-Bridge Cell1/3(si3)
  H-Bridge Driver1/4(4) -> H-Bridge Cell1/4(si4)
  sf23/1 -> H-Bridge Driver2/2(si3)
  sf13/1 -> H-Bridge Driver1/2(si3)
  sf21/1 -> H-Bridge Driver2/1(si1)
  sf31/1 -> H-Bridge Driver3/1(si1)
  sf11/1 -> H-Bridge Driver1/1(si1)
  sf33/1 -> H-Bridge Driver3/2(si3)
  H-Bridge Driver3/2(2) -> H-Bridge Cell3/2(si2)
  H-Bridge Driver3/1(1) -> H-Bridge Cell3/1(si1)
  H-Bridge Driver3/3(3) -> H-Bridge Cell3/3(si3)
  H-Bridge Driver3/4(4) -> H-Bridge Cell3/4(si4)
  connections:
  H-Bridge Cell2/RConn3 -- H-Bridge Cell1/RConn4
  DC-Link2/RConn2 -- H-Bridge Cell2/RConn2
  DC-Link2/RConn1 -- H-Bridge Cell2/RConn1
  H-Bridge Cell1/RConn1 -- DC-Link1/RConn1
  H-Bridge Cell1/RConn2 -- DC-Link1/RConn2
  H-Bridge Cell1/RConn3 -- +/RConn1
  -/RConn1 -- H-Bridge Cell3/RConn4
  H-Bridge Cell3/RConn3 -- H-Bridge Cell2/RConn4
  DC-Link3/RConn2 -- H-Bridge Cell3/RConn2
  DC-Link3/RConn1 -- H-Bridge Cell3/RConn1

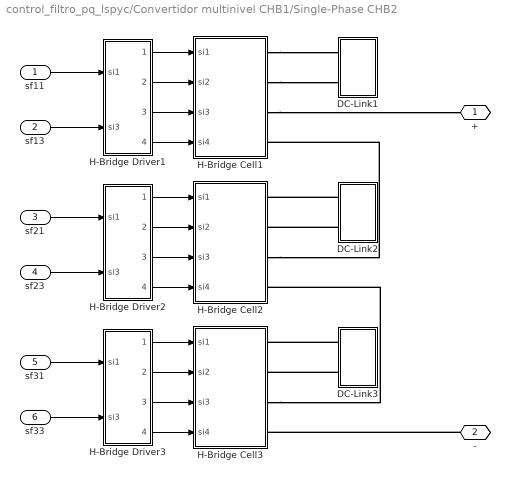
== system control_filtro_pq_lspyc/Convertidor multinivel CHB1/Single-Phase CHB2 ==
  sf11 : Inport
  sf13 : Inport  Port=2
  sf21 : Inport  Port=3
  sf23 : Inport  Port=4
  sf31 : Inport  Port=5
  sf33 : Inport  Port=6
  DC-Link1 : Subsystem
  DC-Link2 : Subsystem
  DC-Link3 : Subsystem
  H-Bridge Cell1 : Subsystem
  H-Bridge Cell2 : Subsystem
  H-Bridge Cell3 : Subsystem
  H-Bridge Driver1 : Subsystem
  H-Bridge Driver2 : Subsystem
  H-Bridge Driver3 : Subsystem
  + : PMIOPort  Port=1  Side=Right
  - : PMIOPort  Port=2  Side=Right
  wires:
  H-Bridge Driver2/1(1) -> H-Bridge Cell2/1(si1)
  H-Bridge Driver2/3(3) -> H-Bridge Cell2/3(si3)
  H-Bridge Driver2/2(2) -> H-Bridge Cell2/2(si2)
  H-Bridge Driver2/4(4) -> H-Bridge Cell2/4(si4)
  H-Bridge Driver1/1(1) -> H-Bridge Cell1/1(si1)
  H-Bridge Driver1/2(2) -> H-Bridge Cell1/2(si2)
  H-Bridge Driver1/3(3) -> H-Bridge Cell1/3(si3)
  H-Bridge Driver1/4(4) -> H-Bridge Cell1/4(si4)
  sf23/1 -> H-Bridge Driver2/2(si3)
  sf13/1 -> H-Bridge Driver1/2(si3)
  sf21/1 -> H-Bridge Driver2/1(si1)
  sf31/1 -> H-Bridge Driver3/1(si1)
  sf11/1 -> H-Bridge Driver1/1(si1)
  sf33/1 -> H-Bridge Driver3/2(si3)
  H-Bridge Driver3/2(2) -> H-Bridge Cell3/2(si2)
  H-Bridge Driver3/1(1) -> H-Bridge Cell3/1(si1)
  H-Bridge Driver3/3(3) -> H-Bridge Cell3/3(si3)
  H-Bridge Driver3/4(4) -> H-Bridge Cell3/4(si4)
  connections:
  H-Bridge Cell2/RConn3 -- H-Bridge Cell1/RConn4
  DC-Link2/RConn2 -- H-Bridge Cell2/RConn2
  DC-Link2/RConn1 -- H-Bridge Cell2/RConn1
  H-Bridge Cell1/RConn1 -- DC-Link1/RConn1
  H-Bridge Cell1/RConn2 -- DC-Link1/RConn2
  H-Bridge Cell1/RConn3 -- +/RConn1
  -/RConn1 -- H-Bridge Cell3/RConn4
  H-Bridge Cell3/RConn3 -- H-Bridge Cell2/RConn4
  DC-Link3/RConn2 -- H-Bridge Cell3/RConn2
  DC-Link3/RConn1 -- H-Bridge Cell3/RConn1

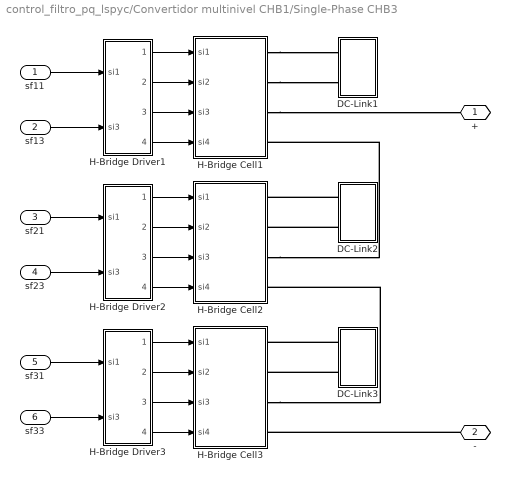
== system control_filtro_pq_lspyc/Convertidor multinivel CHB1/Single-Phase CHB3 ==
  sf11 : Inport
  sf13 : Inport  Port=2
  sf21 : Inport  Port=3
  sf23 : Inport  Port=4
  sf31 : Inport  Port=5
  sf33 : Inport  Port=6
  DC-Link1 : Subsystem
  DC-Link2 : Subsystem
  DC-Link3 : Subsystem
  H-Bridge Cell1 : Subsystem
  H-Bridge Cell2 : Subsystem
  H-Bridge Cell3 : Subsystem
  H-Bridge Driver1 : Subsystem
  H-Bridge Driver2 : Subsystem
  H-Bridge Driver3 : Subsystem
  + : PMIOPort  Port=1  Side=Right
  - : PMIOPort  Port=2  Side=Right
  wires:
  H-Bridge Driver2/1(1) -> H-Bridge Cell2/1(si1)
  H-Bridge Driver2/3(3) -> H-Bridge Cell2/3(si3)
  H-Bridge Driver2/2(2) -> H-Bridge Cell2/2(si2)
  H-Bridge Driver2/4(4) -> H-Bridge Cell2/4(si4)
  H-Bridge Driver1/1(1) -> H-Bridge Cell1/1(si1)
  H-Bridge Driver1/2(2) -> H-Bridge Cell1/2(si2)
  H-Bridge Driver1/3(3) -> H-Bridge Cell1/3(si3)
  H-Bridge Driver1/4(4) -> H-Bridge Cell1/4(si4)
  sf23/1 -> H-Bridge Driver2/2(si3)
  sf13/1 -> H-Bridge Driver1/2(si3)
  sf21/1 -> H-Bridge Driver2/1(si1)
  sf31/1 -> H-Bridge Driver3/1(si1)
  sf11/1 -> H-Bridge Driver1/1(si1)
  sf33/1 -> H-Bridge Driver3/2(si3)
  H-Bridge Driver3/2(2) -> H-Bridge Cell3/2(si2)
  H-Bridge Driver3/1(1) -> H-Bridge Cell3/1(si1)
  H-Bridge Driver3/3(3) -> H-Bridge Cell3/3(si3)
  H-Bridge Driver3/4(4) -> H-Bridge Cell3/4(si4)
  connections:
  H-Bridge Cell2/RConn3 -- H-Bridge Cell1/RConn4
  DC-Link2/RConn2 -- H-Bridge Cell2/RConn2
  DC-Link2/RConn1 -- H-Bridge Cell2/RConn1
  H-Bridge Cell1/RConn1 -- DC-Link1/RConn1
  H-Bridge Cell1/RConn2 -- DC-Link1/RConn2
  H-Bridge Cell1/RConn3 -- +/RConn1
  -/RConn1 -- H-Bridge Cell3/RConn4
  H-Bridge Cell3/RConn3 -- H-Bridge Cell2/RConn4
  DC-Link3/RConn2 -- H-Bridge Cell3/RConn2
  DC-Link3/RConn1 -- H-Bridge Cell3/RConn1

== system control_filtro_pq_lspyc/Phase-Shifted multicarrier modulator/Modulation block a1 ==
  ma : Inport
  Data Type Conversion : DataTypeConversion  OutDataTypeStr=double
  Data Type Conversion3 : DataTypeConversion  OutDataTypeStr=double
  Gain1 : Gain  Gain=-1
  Relational Operator : RelationalOperator  Operator=<=  OutDataTypeStr=boolean  RndMeth=Nearest
  Relational Operator2 : RelationalOperator  Operator=<=  OutDataTypeStr=boolean  RndMeth=Nearest
  Repeating Sequence1 : simulink/Sources/Repeating Sequence  rep_seq_t="[0 (1/fc)/2  1/fc]"  rep_seq_y=[-1 1 -1]
  Scope : Scope
  S1 : Outport
  S3 : Outport  Port=2
  wires:
  Relational Operator/1 -> Data Type Conversion/1
  Repeating Sequence1/1 -> Scope/1, Relational Operator/1, Relational Operator2/1
  Data Type Conversion/1 -> S1/1
  ma/1 -> Relational Operator/2, Gain1/1
  Relational Operator2/1 -> Data Type Conversion3/1
  Data Type Conversion3/1 -> S3/1
  Gain1/1 -> Relational Operator2/2

== system control_filtro_pq_lspyc/Phase-Shifted multicarrier modulator/Modulation block a2 ==
  ma : Inport
  Data Type Conversion : DataTypeConversion  OutDataTypeStr=double
  Data Type Conversion3 : DataTypeConversion  OutDataTypeStr=double
  Gain1 : Gain  Gain=-1
  Relational Operator : RelationalOperator  Operator=<=  OutDataTypeStr=boolean  RndMeth=Nearest
  Relational Operator2 : RelationalOperator  Operator=<=  OutDataTypeStr=boolean  RndMeth=Nearest
  Repeating Sequence1 : simulink/Sources/Repeating Sequence  rep_seq_t="[0 (1/fc)/2  1/fc]"  rep_seq_y=[-1 1 -1]
  Transport Delay : TransportDelay  DelayTime=Tm*(180/nc)/360
  S1 : Outport
  S3 : Outport  Port=2
  wires:
  Relational Operator/1 -> Data Type Conversion/1
  Repeating Sequence1/1 -> Transport Delay/1
  Data Type Conversion/1 -> S1/1
  ma/1 -> Relational Operator/2, Gain1/1
  Relational Operator2/1 -> Data Type Conversion3/1
  Data Type Conversion3/1 -> S3/1
  Gain1/1 -> Relational Operator2/2
  Transport Delay/1 -> Relational Operator/1, Relational Operator2/1

== system control_filtro_pq_lspyc/Phase-Shifted multicarrier modulator/Modulation block a3 ==
  ma : Inport
  Data Type Conversion : DataTypeConversion  OutDataTypeStr=double
  Data Type Conversion3 : DataTypeConversion  OutDataTypeStr=double
  Gain1 : Gain  Gain=-1
  Relational Operator : RelationalOperator  Operator=<=  OutDataTypeStr=boolean  RndMeth=Nearest
  Relational Operator2 : RelationalOperator  Operator=<=  OutDataTypeStr=boolean  RndMeth=Nearest
  Repeating Sequence1 : simulink/Sources/Repeating Sequence  rep_seq_t="[0 (1/fc)/2  1/fc]"  rep_seq_y=[-1 1 -1]
  Transport Delay : TransportDelay  DelayTime=(Tm*(180/nc)/360)*2
  S1 : Outport
  S3 : Outport  Port=2
  wires:
  Relational Operator/1 -> Data Type Conversion/1
  Repeating Sequence1/1 -> Transport Delay/1
  Data Type Conversion/1 -> S1/1
  ma/1 -> Relational Operator/2, Gain1/1
  Relational Operator2/1 -> Data Type Conversion3/1
  Data Type Conversion3/1 -> S3/1
  Gain1/1 -> Relational Operator2/2
  Transport Delay/1 -> Relational Operator/1, Relational Operator2/1

== system control_filtro_pq_lspyc/Phase-Shifted multicarrier modulator/Modulation block b1 ==
  mb : Inport
  Data Type Conversion : DataTypeConversion  OutDataTypeStr=double
  Data Type Conversion3 : DataTypeConversion  OutDataTypeStr=double
  Gain1 : Gain  Gain=-1
  Relational Operator : RelationalOperator  Operator=<=  OutDataTypeStr=boolean  RndMeth=Nearest
  Relational Operator2 : RelationalOperator  Operator=<=  OutDataTypeStr=boolean  RndMeth=Nearest
  Repeating Sequence1 : simulink/Sources/Repeating Sequence  rep_seq_t="[0 (1/fc)/2  1/fc]"  rep_seq_y=[-1 1 -1]
  S1 : Outport
  S3 : Outport  Port=2
  wires:
  Relational Operator/1 -> Data Type Conversion/1
  Repeating Sequence1/1 -> Relational Operator/1, Relational Operator2/1
  Data Type Conversion/1 -> S1/1
  mb/1 -> Relational Operator/2, Gain1/1
  Relational Operator2/1 -> Data Type Conversion3/1
  Data Type Conversion3/1 -> S3/1
  Gain1/1 -> Relational Operator2/2

== system control_filtro_pq_lspyc/Phase-Shifted multicarrier modulator/Modulation block b2 ==
  mb : Inport
  Data Type Conversion : DataTypeConversion  OutDataTypeStr=double
  Data Type Conversion3 : DataTypeConversion  OutDataTypeStr=double
  Gain1 : Gain  Gain=-1
  Relational Operator : RelationalOperator  Operator=<=  OutDataTypeStr=boolean  RndMeth=Nearest
  Relational Operator2 : RelationalOperator  Operator=<=  OutDataTypeStr=boolean  RndMeth=Nearest
  Repeating Sequence1 : simulink/Sources/Repeating Sequence  rep_seq_t="[0 (1/fc)/2  1/fc]"  rep_seq_y=[-1 1 -1]
  Transport Delay : TransportDelay  DelayTime=Tm*(180/nc)/360
  S1 : Outport
  S3 : Outport  Port=2
  wires:
  Relational Operator/1 -> Data Type Conversion/1
  Repeating Sequence1/1 -> Transport Delay/1
  Data Type Conversion/1 -> S1/1
  mb/1 -> Relational Operator/2, Gain1/1
  Relational Operator2/1 -> Data Type Conversion3/1
  Data Type Conversion3/1 -> S3/1
  Gain1/1 -> Relational Operator2/2
  Transport Delay/1 -> Relational Operator/1, Relational Operator2/1

== system control_filtro_pq_lspyc/Phase-Shifted multicarrier modulator/Modulation block b3 ==
  mb : Inport
  Data Type Conversion : DataTypeConversion  OutDataTypeStr=double
  Data Type Conversion3 : DataTypeConversion  OutDataTypeStr=double
  Gain1 : Gain  Gain=-1
  Relational Operator : RelationalOperator  Operator=<=  OutDataTypeStr=boolean  RndMeth=Nearest
  Relational Operator2 : RelationalOperator  Operator=<=  OutDataTypeStr=boolean  RndMeth=Nearest
  Repeating Sequence1 : simulink/Sources/Repeating Sequence  rep_seq_t="[0 (1/fc)/2  1/fc]"  rep_seq_y=[-1 1 -1]
  Transport Delay : TransportDelay  DelayTime=(Tm*(180/nc)/360)*2
  S1 : Outport
  S3 : Outport  Port=2
  wires:
  Relational Operator/1 -> Data Type Conversion/1
  Repeating Sequence1/1 -> Transport Delay/1
  Data Type Conversion/1 -> S1/1
  mb/1 -> Relational Operator/2, Gain1/1
  Relational Operator2/1 -> Data Type Conversion3/1
  Data Type Conversion3/1 -> S3/1
  Gain1/1 -> Relational Operator2/2
  Transport Delay/1 -> Relational Operator/1, Relational Operator2/1

== system control_filtro_pq_lspyc/Phase-Shifted multicarrier modulator/Modulation block b4 ==
  mb : Inport
  Data Type Conversion : DataTypeConversion  OutDataTypeStr=double
  Data Type Conversion3 : DataTypeConversion  OutDataTypeStr=double
  Gain1 : Gain  Gain=-1
  Relational Operator : RelationalOperator  Operator=<=  OutDataTypeStr=boolean  RndMeth=Nearest
  Relational Operator2 : RelationalOperator  Operator=<=  OutDataTypeStr=boolean  RndMeth=Nearest
  Repeating Sequence1 : simulink/Sources/Repeating Sequence  rep_seq_t="[0 (1/fc)/2  1/fc]"  rep_seq_y=[-1 1 -1]
  S1 : Outport
  S3 : Outport  Port=2
  wires:
  Relational Operator/1 -> Data Type Conversion/1
  Repeating Sequence1/1 -> Relational Operator/1, Relational Operator2/1
  Data Type Conversion/1 -> S1/1
  mb/1 -> Relational Operator/2, Gain1/1
  Relational Operator2/1 -> Data Type Conversion3/1
  Data Type Conversion3/1 -> S3/1
  Gain1/1 -> Relational Operator2/2

== system control_filtro_pq_lspyc/Phase-Shifted multicarrier modulator/Modulation block b5 ==
  mb : Inport
  Data Type Conversion : DataTypeConversion  OutDataTypeStr=double
  Data Type Conversion3 : DataTypeConversion  OutDataTypeStr=double
  Gain1 : Gain  Gain=-1
  Relational Operator : RelationalOperator  Operator=<=  OutDataTypeStr=boolean  RndMeth=Nearest
  Relational Operator2 : RelationalOperator  Operator=<=  OutDataTypeStr=boolean  RndMeth=Nearest
  Repeating Sequence1 : simulink/Sources/Repeating Sequence  rep_seq_t="[0 (1/fc)/2  1/fc]"  rep_seq_y=[-1 1 -1]
  Transport Delay : TransportDelay  DelayTime=Tm*(180/nc)/360
  S1 : Outport
  S3 : Outport  Port=2
  wires:
  Relational Operator/1 -> Data Type Conversion/1
  Repeating Sequence1/1 -> Transport Delay/1
  Data Type Conversion/1 -> S1/1
  mb/1 -> Relational Operator/2, Gain1/1
  Relational Operator2/1 -> Data Type Conversion3/1
  Data Type Conversion3/1 -> S3/1
  Gain1/1 -> Relational Operator2/2
  Transport Delay/1 -> Relational Operator/1, Relational Operator2/1

== system control_filtro_pq_lspyc/Phase-Shifted multicarrier modulator/Modulation block b6 ==
  mb : Inport
  Data Type Conversion : DataTypeConversion  OutDataTypeStr=double
  Data Type Conversion3 : DataTypeConversion  OutDataTypeStr=double
  Gain1 : Gain  Gain=-1
  Relational Operator : RelationalOperator  Operator=<=  OutDataTypeStr=boolean  RndMeth=Nearest
  Relational Operator2 : RelationalOperator  Operator=<=  OutDataTypeStr=boolean  RndMeth=Nearest
  Repeating Sequence1 : simulink/Sources/Repeating Sequence  rep_seq_t="[0 (1/fc)/2  1/fc]"  rep_seq_y=[-1 1 -1]
  Transport Delay : TransportDelay  DelayTime=(Tm*(180/nc)/360)*2
  S1 : Outport
  S3 : Outport  Port=2
  wires:
  Relational Operator/1 -> Data Type Conversion/1
  Repeating Sequence1/1 -> Transport Delay/1
  Data Type Conversion/1 -> S1/1
  mb/1 -> Relational Operator/2, Gain1/1
  Relational Operator2/1 -> Data Type Conversion3/1
  Data Type Conversion3/1 -> S3/1
  Gain1/1 -> Relational Operator2/2
  Transport Delay/1 -> Relational Operator/1, Relational Operator2/1

== system control_filtro_pq_lspyc/Convertidor multinivel CHB1/Single-Phase CHB1/DC-Link1 ==
  Constant : Constant  Value=Ideal
  DC Capacitor : powerlib/Elements/Series RLC Branch  LConnTagsString=__new0  RConnTagsString=__new0  BranchType=C  Resistance=0.09  Inductance=0.002996  SetiL0=off  InitialCurrent=0  Capacitance=Cdc  Setx0=on  InitialVoltage=Vodc  Measurements=None
  DC Voltage Source : powerlib/Electrical Sources/DC Voltage Source  Amplitude=Vdc  Measurements=None
  Ideal Switch : powerlib/Power Electronics/Ideal Switch  Ron=0.001  Lon=0  IC=0  Rs=1e5  Cs=inf  Measurements=off
  Ideal Switch2 : powerlib/Power Electronics/Ideal Switch  Ron=0.001  Lon=0  IC=0  Rs=1e5  Cs=inf  Measurements=off
  Logical Operator2 : Logic  Operator=NOT  AllPortsSameDT=off  OutDataTypeStr=boolean
  Vcan3 : powerlib/Measurements/Voltage Measurement  PhasorSimulation=off  OutputType=Complex  PSBequivalent=0
  + : PMIOPort  Port=1  Side=Right
  - : PMIOPort  Port=2  Side=Right
  tag scope: Vcca1=global
  wires:
  Constant/1 -> Ideal Switch/1, Logical Operator2/1
  Logical Operator2/1 -> Ideal Switch2/1
  Vcan3/1 -> [Vcca1]
  connections:
  Ideal Switch/RConn1 -- Ideal Switch2/RConn1 -- Vcan3/LConn1 -- +/RConn1
  DC Voltage Source/RConn1 -- Ideal Switch/LConn1
  -/RConn1 -- Vcan3/LConn2 -- DC Voltage Source/LConn1 -- DC Capacitor/RConn1
  Ideal Switch2/LConn1 -- DC Capacitor/LConn1

== system control_filtro_pq_lspyc/Convertidor multinivel CHB1/Single-Phase CHB1/DC-Link2 ==
  Constant : Constant  Value=Ideal
  DC Capacitor : powerlib/Elements/Series RLC Branch  LConnTagsString=__new0  RConnTagsString=__new0  BranchType=C  Resistance=0.09  Inductance=0.002996  SetiL0=off  InitialCurrent=0  Capacitance=Cdc  Setx0=on  InitialVoltage=Vodc  Measurements=None
  DC Voltage Source : powerlib/Electrical Sources/DC Voltage Source  Amplitude=Vdc  Measurements=None
  Ideal Switch : powerlib/Power Electronics/Ideal Switch  Ron=0.001  Lon=0  IC=0  Rs=1e5  Cs=inf  Measurements=off
  Ideal Switch2 : powerlib/Power Electronics/Ideal Switch  Ron=0.001  Lon=0  IC=0  Rs=1e5  Cs=inf  Measurements=off
  Logical Operator2 : Logic  Operator=NOT  AllPortsSameDT=off  OutDataTypeStr=boolean
  Vcan3 : powerlib/Measurements/Voltage Measurement  PhasorSimulation=off  OutputType=Complex  PSBequivalent=0
  + : PMIOPort  Port=1  Side=Right
  - : PMIOPort  Port=2  Side=Right
  tag scope: Vcca2=global
  wires:
  Constant/1 -> Ideal Switch/1, Logical Operator2/1
  Logical Operator2/1 -> Ideal Switch2/1
  Vcan3/1 -> [Vcca2]
  connections:
  Ideal Switch/RConn1 -- Ideal Switch2/RConn1 -- Vcan3/LConn1 -- +/RConn1
  DC Voltage Source/RConn1 -- Ideal Switch/LConn1
  -/RConn1 -- DC Capacitor/RConn1 -- DC Voltage Source/LConn1 -- Vcan3/LConn2
  Ideal Switch2/LConn1 -- DC Capacitor/LConn1

== system control_filtro_pq_lspyc/Convertidor multinivel CHB1/Single-Phase CHB1/DC-Link3 ==
  Constant : Constant  Value=Ideal
  DC Capacitor : powerlib/Elements/Series RLC Branch  LConnTagsString=__new0  RConnTagsString=__new0  BranchType=C  Resistance=0.09  Inductance=0.002996  SetiL0=off  InitialCurrent=0  Capacitance=Cdc  Setx0=on  InitialVoltage=Vodc  Measurements=None
  DC Voltage Source : powerlib/Electrical Sources/DC Voltage Source  Amplitude=Vdc  Measurements=None
  Ideal Switch : powerlib/Power Electronics/Ideal Switch  Ron=0.001  Lon=0  IC=0  Rs=1e5  Cs=inf  Measurements=off
  Ideal Switch2 : powerlib/Power Electronics/Ideal Switch  Ron=0.001  Lon=0  IC=0  Rs=1e5  Cs=inf  Measurements=off
  Logical Operator2 : Logic  Operator=NOT  AllPortsSameDT=off  OutDataTypeStr=boolean
  Vcan3 : powerlib/Measurements/Voltage Measurement  PhasorSimulation=off  OutputType=Complex  PSBequivalent=0
  + : PMIOPort  Port=1  Side=Right
  - : PMIOPort  Port=2  Side=Right
  tag scope: Vcca3=global
  wires:
  Constant/1 -> Ideal Switch/1, Logical Operator2/1
  Logical Operator2/1 -> Ideal Switch2/1
  Vcan3/1 -> [Vcca3]
  connections:
  Ideal Switch/RConn1 -- Ideal Switch2/RConn1 -- Vcan3/LConn1 -- +/RConn1
  DC Voltage Source/RConn1 -- Ideal Switch/LConn1
  -/RConn1 -- Vcan3/LConn2 -- DC Capacitor/RConn1 -- DC Voltage Source/LConn1
  DC Capacitor/LConn1 -- Ideal Switch2/LConn1

== system control_filtro_pq_lspyc/Convertidor multinivel CHB1/Single-Phase CHB1/H-Bridge Cell1 ==
  si1 : Inport
  si2 : Inport  Port=2
  si3 : Inport  Port=3
  si4 : Inport  Port=4
  IGBT/Diode{1..4} (4 alike) : powerlib/Power Electronics/IGBT//Diode  Ron=Ron  Rs=Rs  Cs=Cs  Measurements=off
  DC+ : PMIOPort  Port=1  Side=Right
  DC- : PMIOPort  Port=2  Side=Right
  + : PMIOPort  Port=3  Side=Right
  - : PMIOPort  Port=4  Side=Right
  wires:
  si4/1 -> IGBT/Diode4/1
  si2/1 -> IGBT/Diode2/1
  si3/1 -> IGBT/Diode3/1
  si1/1 -> IGBT/Diode1/1
  connections:
  IGBT/Diode3/RConn1 -- IGBT/Diode4/LConn1 -- -/RConn1
  DC-/RConn1 -- IGBT/Diode4/RConn1 -- IGBT/Diode2/RConn1
  IGBT/Diode1/RConn1 -- IGBT/Diode2/LConn1 -- +/RConn1
  IGBT/Diode1/LConn1 -- IGBT/Diode3/LConn1 -- DC+/RConn1

== system control_filtro_pq_lspyc/Convertidor multinivel CHB1/Single-Phase CHB1/H-Bridge Cell2 ==
  si1 : Inport
  si2 : Inport  Port=2
  si3 : Inport  Port=3
  si4 : Inport  Port=4
  IGBT/Diode{1..4} (4 alike) : powerlib/Power Electronics/IGBT//Diode  Ron=Ron  Rs=Rs  Cs=Cs  Measurements=off
  DC+ : PMIOPort  Port=1  Side=Right
  DC- : PMIOPort  Port=2  Side=Right
  + : PMIOPort  Port=3  Side=Right
  - : PMIOPort  Port=4  Side=Right
  wires:
  si4/1 -> IGBT/Diode4/1
  si2/1 -> IGBT/Diode2/1
  si3/1 -> IGBT/Diode3/1
  si1/1 -> IGBT/Diode1/1
  connections:
  IGBT/Diode3/RConn1 -- IGBT/Diode4/LConn1 -- -/RConn1
  IGBT/Diode2/RConn1 -- IGBT/Diode4/RConn1 -- DC-/RConn1
  IGBT/Diode1/RConn1 -- IGBT/Diode2/LConn1 -- +/RConn1
  IGBT/Diode1/LConn1 -- IGBT/Diode3/LConn1 -- DC+/RConn1

== system control_filtro_pq_lspyc/Convertidor multinivel CHB1/Single-Phase CHB1/H-Bridge Cell3 ==
  si1 : Inport
  si2 : Inport  Port=2
  si3 : Inport  Port=3
  si4 : Inport  Port=4
  IGBT/Diode{1..4} (4 alike) : powerlib/Power Electronics/IGBT//Diode  Ron=Ron  Rs=Rs  Cs=Cs  Measurements=off
  DC+ : PMIOPort  Port=1  Side=Right
  DC- : PMIOPort  Port=2  Side=Right
  + : PMIOPort  Port=3  Side=Right
  - : PMIOPort  Port=4  Side=Right
  wires:
  si4/1 -> IGBT/Diode4/1
  si2/1 -> IGBT/Diode2/1
  si3/1 -> IGBT/Diode3/1
  si1/1 -> IGBT/Diode1/1
  connections:
  IGBT/Diode3/RConn1 -- IGBT/Diode4/LConn1 -- -/RConn1
  IGBT/Diode2/RConn1 -- IGBT/Diode4/RConn1 -- DC-/RConn1
  IGBT/Diode1/RConn1 -- IGBT/Diode2/LConn1 -- +/RConn1
  IGBT/Diode1/LConn1 -- IGBT/Diode3/LConn1 -- DC+/RConn1

== system control_filtro_pq_lspyc/Convertidor multinivel CHB1/Single-Phase CHB1/H-Bridge Driver1 ==
  si1 : Inport
  si3 : Inport  Port=2
  Logical Operator2 : Logic  Operator=NOT  AllPortsSameDT=off  OutDataTypeStr=boolean
  Logical Operator3 : Logic  Operator=NOT  AllPortsSameDT=off  OutDataTypeStr=boolean
  1 : Outport
  2 : Outport  Port=2
  3 : Outport  Port=3
  4 : Outport  Port=4
  wires:
  si3/1 -> 3/1, Logical Operator3/1
  si1/1 -> 1/1, Logical Operator2/1
  Logical Operator3/1 -> 4/1
  Logical Operator2/1 -> 2/1

== system control_filtro_pq_lspyc/Convertidor multinivel CHB1/Single-Phase CHB1/H-Bridge Driver2 ==
  si1 : Inport
  si3 : Inport  Port=2
  Logical Operator2 : Logic  Operator=NOT  AllPortsSameDT=off  OutDataTypeStr=boolean
  Logical Operator3 : Logic  Operator=NOT  AllPortsSameDT=off  OutDataTypeStr=boolean
  1 : Outport
  2 : Outport  Port=2
  3 : Outport  Port=3
  4 : Outport  Port=4
  wires:
  si3/1 -> 3/1, Logical Operator3/1
  si1/1 -> 1/1, Logical Operator2/1
  Logical Operator3/1 -> 4/1
  Logical Operator2/1 -> 2/1

== system control_filtro_pq_lspyc/Convertidor multinivel CHB1/Single-Phase CHB1/H-Bridge Driver3 ==
  si1 : Inport
  si3 : Inport  Port=2
  Logical Operator2 : Logic  Operator=NOT  AllPortsSameDT=off  OutDataTypeStr=boolean
  Logical Operator3 : Logic  Operator=NOT  AllPortsSameDT=off  OutDataTypeStr=boolean
  1 : Outport
  2 : Outport  Port=2
  3 : Outport  Port=3
  4 : Outport  Port=4
  wires:
  si3/1 -> 3/1, Logical Operator3/1
  si1/1 -> 1/1, Logical Operator2/1
  Logical Operator3/1 -> 4/1
  Logical Operator2/1 -> 2/1

== system control_filtro_pq_lspyc/Convertidor multinivel CHB1/Single-Phase CHB2/DC-Link1 ==
  Constant : Constant  Value=Ideal
  DC Capacitor : powerlib/Elements/Series RLC Branch  LConnTagsString=__new0  RConnTagsString=__new0  BranchType=C  Resistance=0.09  Inductance=0.002996  SetiL0=off  InitialCurrent=0  Capacitance=Cdc  Setx0=on  InitialVoltage=Vodc  Measurements=None
  DC Voltage Source : powerlib/Electrical Sources/DC Voltage Source  Amplitude=Vdc  Measurements=None
  Ideal Switch : powerlib/Power Electronics/Ideal Switch  Ron=0.001  Lon=0  IC=0  Rs=1e5  Cs=inf  Measurements=off
  Ideal Switch2 : powerlib/Power Electronics/Ideal Switch  Ron=0.001  Lon=0  IC=0  Rs=1e5  Cs=inf  Measurements=off
  Logical Operator2 : Logic  Operator=NOT  AllPortsSameDT=off  OutDataTypeStr=boolean
  Vcan3 : powerlib/Measurements/Voltage Measurement  PhasorSimulation=off  OutputType=Complex  PSBequivalent=0
  + : PMIOPort  Port=1  Side=Right
  - : PMIOPort  Port=2  Side=Right
  tag scope: Vccb1=global
  wires:
  Constant/1 -> Ideal Switch/1, Logical Operator2/1
  Logical Operator2/1 -> Ideal Switch2/1
  Vcan3/1 -> [Vccb1]
  connections:
  Ideal Switch/RConn1 -- Ideal Switch2/RConn1 -- Vcan3/LConn1 -- +/RConn1
  DC Voltage Source/RConn1 -- Ideal Switch/LConn1
  -/RConn1 -- Vcan3/LConn2 -- DC Voltage Source/LConn1 -- DC Capacitor/RConn1
  Ideal Switch2/LConn1 -- DC Capacitor/LConn1

== system control_filtro_pq_lspyc/Convertidor multinivel CHB1/Single-Phase CHB2/DC-Link2 ==
  Constant : Constant  Value=Ideal
  DC Capacitor : powerlib/Elements/Series RLC Branch  LConnTagsString=__new0  RConnTagsString=__new0  BranchType=C  Resistance=0.09  Inductance=0.002996  SetiL0=off  InitialCurrent=0  Capacitance=Cdc  Setx0=on  InitialVoltage=Vodc  Measurements=None
  DC Voltage Source : powerlib/Electrical Sources/DC Voltage Source  Amplitude=Vdc  Measurements=None
  Ideal Switch : powerlib/Power Electronics/Ideal Switch  Ron=0.001  Lon=0  IC=0  Rs=1e5  Cs=inf  Measurements=off
  Ideal Switch2 : powerlib/Power Electronics/Ideal Switch  Ron=0.001  Lon=0  IC=0  Rs=1e5  Cs=inf  Measurements=off
  Logical Operator2 : Logic  Operator=NOT  AllPortsSameDT=off  OutDataTypeStr=boolean
  Vcan3 : powerlib/Measurements/Voltage Measurement  PhasorSimulation=off  OutputType=Complex  PSBequivalent=0
  + : PMIOPort  Port=1  Side=Right
  - : PMIOPort  Port=2  Side=Right
  tag scope: Vccb2=global
  wires:
  Constant/1 -> Ideal Switch/1, Logical Operator2/1
  Vcan3/1 -> [Vccb2]
  Logical Operator2/1 -> Ideal Switch2/1
  connections:
  Ideal Switch/RConn1 -- Ideal Switch2/RConn1 -- Vcan3/LConn1 -- +/RConn1
  DC Voltage Source/RConn1 -- Ideal Switch/LConn1
  -/RConn1 -- DC Capacitor/RConn1 -- DC Voltage Source/LConn1 -- Vcan3/LConn2
  Ideal Switch2/LConn1 -- DC Capacitor/LConn1
